simulink model "Scenario_2_power_system_modeling"  (R2023b)
settings: Solver=ode4  StartTime=0.0  StopTime=90  FixedStep=0.01  RelTol=1e-3
values from neighbouring files (symbols this model uses):
  a12 = -1    [simulation_3_Area_scenario.m]    (also in simulation_scenario_1_2_3.m)
  B1 = (1/Rtotal_1) + D1    (= 20.9)    [simulation_3_Area_scenario.m]    (also in simulation_scenario_1_2_3.m = 40.9)
  B2 = (1/Rtotal_2) + D2    (= 21.5)    [simulation_3_Area_scenario.m]    (also in simulation_scenario_1_2_3.m = 41.5)
  D1 = 0.9    [simulation_3_Area_scenario.m]    (also in simulation_scenario_1_2_3.m)
  D2 = 1.5    [simulation_3_Area_scenario.m]    (also in simulation_scenario_1_2_3.m)
  Fhp = 0.4    [simulation_3_Area_scenario.m]    (also in simulation_scenario_1_2_3.m)
  H1 = H1_values(i)    [simulation_3_Area_scenario.m]    (also in simulation_scenario_1_2_3.m)
  H2 = H2_values(i)    [simulation_3_Area_scenario.m]    (also in simulation_scenario_1_2_3.m)
  KI1 = 0.25    [simulation_3_Area_scenario.m]    (also in simulation_scenario_1_2_3.m)
  KI2 = 0.25    [simulation_3_Area_scenario.m]    (also in simulation_scenario_1_2_3.m)
  KI3 = 0.25    [simulation_3_Area_scenario.m]    (also in simulation_scenario_1_2_3.m)
  KI4 = 0.25    [simulation_3_Area_scenario.m]    (also in simulation_scenario_1_2_3.m)
  R1 = 0.1    [simulation_3_Area_scenario.m]    (also in simulation_scenario_1_2_3.m = 0.05)
  R2 = 0.1    [simulation_3_Area_scenario.m]    (also in simulation_scenario_1_2_3.m = 0.05)
  R3 = 0.1    [simulation_3_Area_scenario.m]    (also in simulation_scenario_1_2_3.m = 0.05)
  R4 = 0.1    [simulation_3_Area_scenario.m]    (also in simulation_scenario_1_2_3.m = 0.05)
  Rp = 0.05    [simulation_3_Area_scenario.m]    (also in simulation_scenario_1_2_3.m)
  Rt = 0.38    [simulation_3_Area_scenario.m]    (also in simulation_scenario_1_2_3.m)
  T12 = 2    [simulation_3_Area_scenario.m]    (also in simulation_scenario_1_2_3.m)
  Tch1 = 0.39    [simulation_3_Area_scenario.m]    (also in simulation_scenario_1_2_3.m)
  Tch2 = 0.5    [simulation_3_Area_scenario.m]    (also in simulation_scenario_1_2_3.m)
  Tg1 = 0.23    [simulation_3_Area_scenario.m]    (also in simulation_scenario_1_2_3.m)
  Tg2 = 0.14    [simulation_3_Area_scenario.m]    (also in simulation_scenario_1_2_3.m)
  Tg3 = 0.4    [simulation_3_Area_scenario.m]    (also in simulation_scenario_1_2_3.m)
  Tg4 = 0.3    [simulation_3_Area_scenario.m]    (also in simulation_scenario_1_2_3.m)
  Tr = 5    [simulation_3_Area_scenario.m]    (also in simulation_scenario_1_2_3.m)
  Trh = 7    [simulation_3_Area_scenario.m]    (also in simulation_scenario_1_2_3.m)
  Tw = 2.25    [simulation_3_Area_scenario.m]    (also in simulation_scenario_1_2_3.m)
libraries: dspfdesign x2, simulink x2
settings Model: Creator=themi  LastModifiedBy=themi

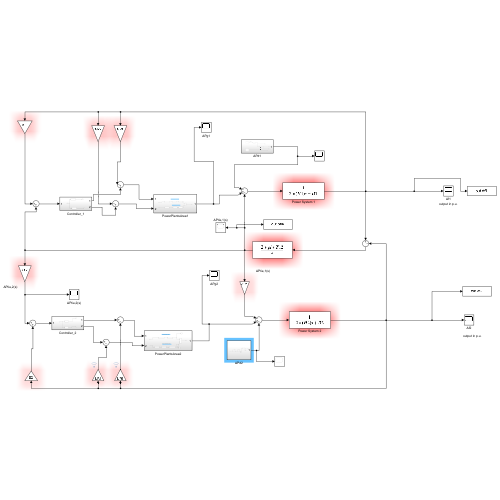
[thumbnail: Simulink's stored preview of the top-level diagram]
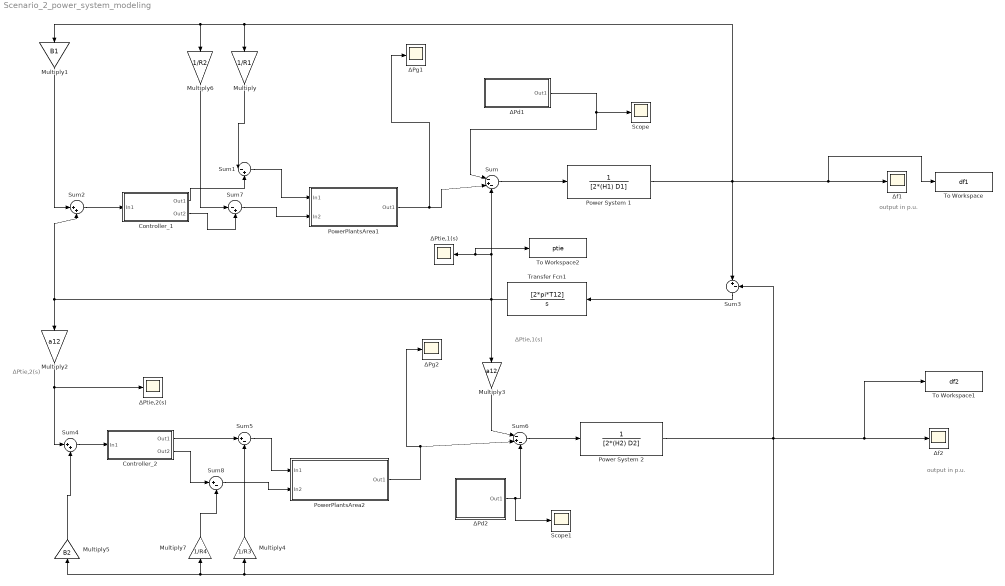
== system Scenario_2_power_system_modeling ==
  note: output in p.u.
  note: output in p.u.
  note: ΔPtie,1(s)
  note: ΔPtie,2(s)
  Controller_1 : Subsystem
  Controller_2 : Subsystem
  Multiply : Gain  Gain=1/R1
  Multiply1 : Gain  Gain=B1
  Multiply2 : Gain  Gain=a12
  Multiply3 : Gain  Gain=a12
  Multiply4 : Gain  Gain=1/R3
  Multiply5 : Gain  Gain=B2
  Multiply6 : Gain  Gain=1/R2
  Multiply7 : Gain  Gain=1/R4
  Power System 1 : TransferFcn  Denominator=[2*(H1) D1]
  Power System 2 : TransferFcn  Denominator=[2*(H2) D2]
  PowerPlantsArea1 : Subsystem
  PowerPlantsArea2 : Subsystem
  Scope : Scope
  Scope1 : Scope
  Sum : Sum  Inputs=|-+-
  Sum1 : Sum  Inputs=|-+
  Sum2 : Sum  Inputs=|++
  Sum3 : Sum  Inputs=|+-
  Sum4 : Sum  Inputs=|++
  Sum5 : Sum  Inputs=|+-
  Sum6 : Sum  Inputs=|-+-
  Sum7 : Sum  Inputs=|-+
  Sum8 : Sum  Inputs=|+-
  To Workspace : ToWorkspace  VariableName=df1  SaveFormat=Structure With Time  SampleTime=-1
  To Workspace1 : ToWorkspace  VariableName=df2  SaveFormat=Structure With Time  SampleTime=-1
  To Workspace2 : ToWorkspace  VariableName=ptie  SaveFormat=Structure With Time  SampleTime=-1
  Transfer Fcn1 : TransferFcn  Numerator=[2*pi*T12]  Denominator=[1 0]
  ΔPd1 : Subsystem
  ΔPd2 : Subsystem
  ΔPg1 : Scope
  ΔPg2 : Scope
  ΔPtie,1(s) : Scope
  ΔPtie,2(s) : Scope
  Δf1 : Scope
  Δf2 : Scope
  wires:
  Sum3/1 -> Transfer Fcn1/1
  Multiply5/1 -> Sum4/2
  Sum/1 -> Power System 1/1
  Multiply4/1 -> Sum5/2
  Sum6/1 -> Power System 2/1
  Sum4/1 -> Controller_2/1(In1)
  Multiply7/1 -> Sum8/2
  Power System 1/1 -> Multiply6/1, Multiply1/1, Multiply/1, To Workspace/1, Δf1/1, Sum3/1
  Multiply3/1 -> Sum6/1
  Sum2/1 -> Controller_1/1(In1)
  Power System 2/1 -> To Workspace1/1, Δf2/1, Multiply7/1, Multiply5/1, Multiply4/1, Sum3/2
  Multiply2/1 -> ΔPtie,2(s)/1, Sum4/1
  Multiply1/1 -> Sum2/1
  Controller_2/1(Out1) -> Sum5/1
  Transfer Fcn1/1 -> Sum2/2, Multiply2/1, Multiply3/1, To Workspace2/1, ΔPtie,1(s)/1, Sum/3
  Multiply/1 -> Sum1/1
  Controller_2/2(Out2) -> Sum8/1
  Controller_1/2(Out2) -> Sum7/2
  Controller_1/1(Out1) -> Sum1/2
  Multiply6/1 -> Sum7/1
  Sum5/1 -> PowerPlantsArea2/1(In1)
  Sum8/1 -> PowerPlantsArea2/2(In2)
  PowerPlantsArea2/1(Out1) -> Sum6/2, ΔPg2/1
  Sum1/1 -> PowerPlantsArea1/1(In1)
  Sum7/1 -> PowerPlantsArea1/2(In2)
  PowerPlantsArea1/1(Out1) -> ΔPg1/1, Sum/2
  ΔPd1/1(Out1) -> Scope/1, Sum/1
  ΔPd2/1(Out1) -> Scope1/1, Sum6/3

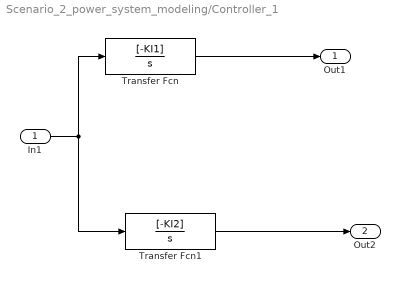
== system Scenario_2_power_system_modeling/Controller_1 ==
  In1 : Inport
  Transfer Fcn : TransferFcn  Numerator=[-KI1]  Denominator=[1 0]
  Transfer Fcn1 : TransferFcn  Numerator=[-KI2]  Denominator=[1 0]
  Out1 : Outport
  Out2 : Outport  Port=2
  wires:
  In1/1 -> Transfer Fcn/1, Transfer Fcn1/1
  Transfer Fcn/1 -> Out1/1
  Transfer Fcn1/1 -> Out2/1

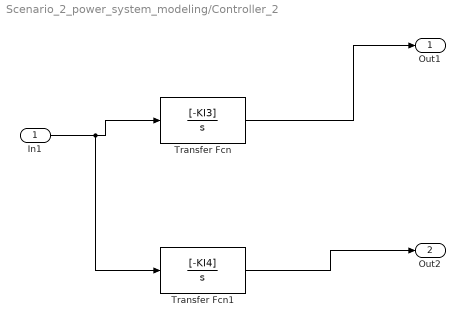
== system Scenario_2_power_system_modeling/Controller_2 ==
  In1 : Inport
  Transfer Fcn : TransferFcn  Numerator=[-KI3]  Denominator=[1 0]
  Transfer Fcn1 : TransferFcn  Numerator=[-KI4]  Denominator=[1 0]
  Out1 : Outport
  Out2 : Outport  Port=2
  wires:
  In1/1 -> Transfer Fcn1/1, Transfer Fcn/1
  Transfer Fcn/1 -> Out1/1
  Transfer Fcn1/1 -> Out2/1

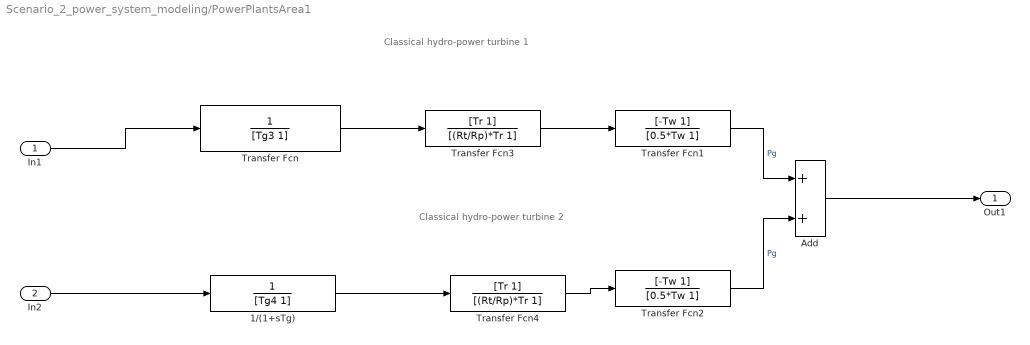
== system Scenario_2_power_system_modeling/PowerPlantsArea1 ==
  note: Classical hydro-power turbine 1
  note: Classical hydro-power turbine 2
  In1 : Inport
  In2 : Inport  Port=2
  1/(1+sTg) : TransferFcn  Denominator=[Tg4 1]
  Add : Sum
  Transfer Fcn : TransferFcn  Denominator=[Tg3 1]
  Transfer Fcn1 : TransferFcn  Numerator=[-Tw 1]  Denominator=[0.5*Tw 1]
  Transfer Fcn2 : TransferFcn  Numerator=[-Tw 1]  Denominator=[0.5*Tw 1]
  Transfer Fcn3 : TransferFcn  Numerator=[Tr 1]  Denominator=[(Rt/Rp)*Tr 1]
  Transfer Fcn4 : TransferFcn  Numerator=[Tr 1]  Denominator=[(Rt/Rp)*Tr 1]
  Out1 : Outport
  wires:
  Transfer Fcn3/1 -> Transfer Fcn1/1
  Transfer Fcn1/1 -> Add/1  "Pg"
  Transfer Fcn/1 -> Transfer Fcn3/1
  In1/1 -> Transfer Fcn/1
  Add/1 -> Out1/1
  In2/1 -> 1/(1+sTg)/1
  Transfer Fcn4/1 -> Transfer Fcn2/1
  1/(1+sTg)/1 -> Transfer Fcn4/1
  Transfer Fcn2/1 -> Add/2  "Pg"

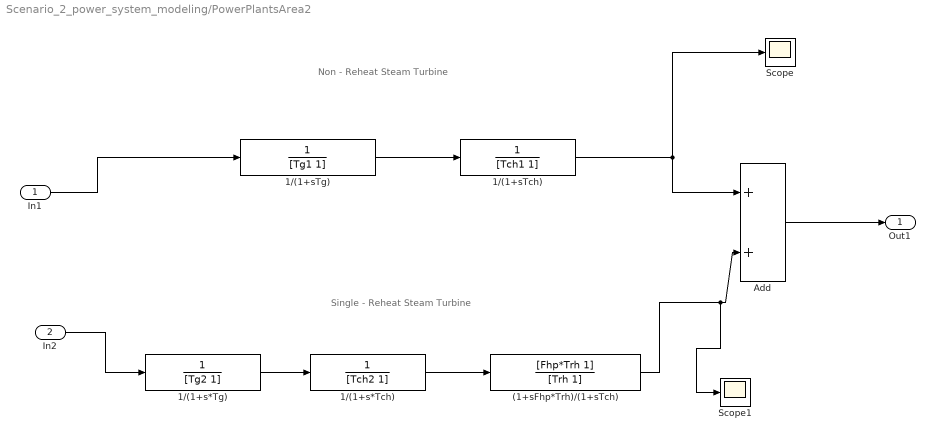
== system Scenario_2_power_system_modeling/PowerPlantsArea2 ==
  note: Non - Reheat Steam Turbine
  note: Single - Reheat Steam Turbine
  In1 : Inport
  In2 : Inport  Port=2
  (1+sFhp*Trh)/(1+sTch) : TransferFcn  Numerator=[Fhp*Trh 1]  Denominator=[Trh 1]
  1/(1+s*Tch) : TransferFcn  Denominator=[Tch2 1]
  1/(1+s*Tg) : TransferFcn  Denominator=[Tg2 1]
  1/(1+sTch) : TransferFcn  Denominator=[Tch1 1]
  1/(1+sTg) : TransferFcn  Denominator=[Tg1 1]
  Add : Sum
  Scope : Scope
  Scope1 : Scope
  Out1 : Outport
  wires:
  In1/1 -> 1/(1+sTg)/1
  1/(1+sTg)/1 -> 1/(1+sTch)/1
  1/(1+s*Tg)/1 -> 1/(1+s*Tch)/1
  1/(1+s*Tch)/1 -> (1+sFhp*Trh)/(1+sTch)/1
  Add/1 -> Out1/1
  1/(1+sTch)/1 -> Scope/1, Add/1
  (1+sFhp*Trh)/(1+sTch)/1 -> Scope1/1, Add/2
  In2/1 -> 1/(1+s*Tg)/1

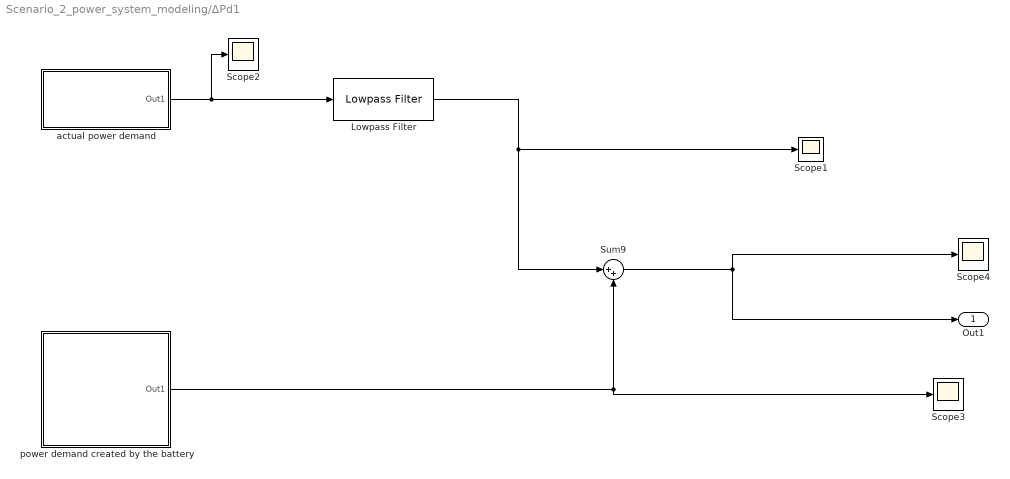
== system Scenario_2_power_system_modeling/ΔPd1 ==
  Lowpass Filter : dspfdesign/Lowpass Filter  FilterType=FIR  DesignForMinimumOrder=on  FilterOrder=50  PassbandFrequency=1  StopbandFrequency=5  PassbandRipple=0.1  StopbandAttenuation=80  SampleRateMode=Specify on dialog  SampleRate=100  SimulateUsing=Interpreted execution  roundingMode=Floor  coeffsDataTypeStr=fixdt(1,16)
  Scope{1..4} (4 alike) : Scope
  Sum9 : Sum  Inputs=|++
  actual power demand : Subsystem
  power demand created by the battery : Subsystem
      mask Display: image('5998565.png');
  Out1 : Outport
  wires:
  Sum9/1 -> Scope4/1, Out1/1
  power demand created by the battery/1(Out1) -> Scope3/1, Sum9/2
  actual power demand/1(Out1) -> Scope2/1, Lowpass Filter/1
  Lowpass Filter/1 -> Scope1/1, Sum9/1

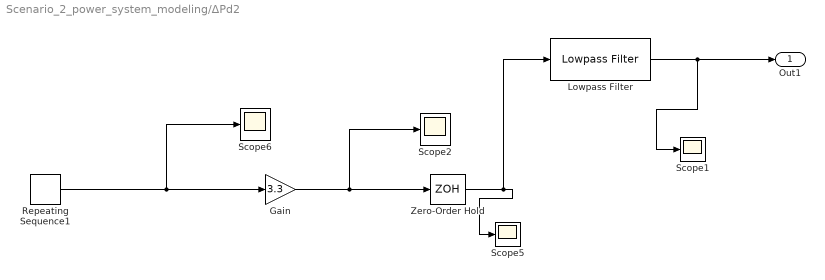
== system Scenario_2_power_system_modeling/ΔPd2 ==
  Gain : Gain  Gain=3.3
  Lowpass Filter : dspfdesign/Lowpass Filter  FilterType=FIR  DesignForMinimumOrder=on  FilterOrder=50  PassbandFrequency=1  StopbandFrequency=5  PassbandRipple=0.1  StopbandAttenuation=80  SampleRateMode=Specify on dialog  SampleRate=100  SimulateUsing=Interpreted execution  roundingMode=Floor  coeffsDataTypeStr=fixdt(1,16)
  Repeating Sequence1 : simulink/Sources/Repeating Sequence  rep_seq_t=t  rep_seq_y=disturbance2
  Scope{1..2,5..6} (4 alike) : Scope
  Zero-Order Hold : ZeroOrderHold  SampleTime=0.01
  Out1 : Outport
  wires:
  Gain/1 -> Scope2/1, Zero-Order Hold/1
  Zero-Order Hold/1 -> Lowpass Filter/1, Scope5/1
  Repeating Sequence1/1 -> Scope6/1, Gain/1
  Lowpass Filter/1 -> Scope1/1, Out1/1

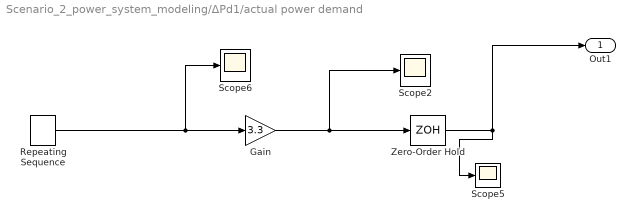
== system Scenario_2_power_system_modeling/ΔPd1/actual power demand ==
  Gain : Gain  Gain=3.3
  Repeating Sequence : simulink/Sources/Repeating Sequence  rep_seq_t=t  rep_seq_y=disturbance1
  Scope2 : Scope
  Scope5 : Scope
  Scope6 : Scope
  Zero-Order Hold : ZeroOrderHold  SampleTime=0.01
  Out1 : Outport
  wires:
  Gain/1 -> Scope2/1, Zero-Order Hold/1
  Repeating Sequence/1 -> Scope6/1, Gain/1
  Zero-Order Hold/1 -> Out1/1, Scope5/1

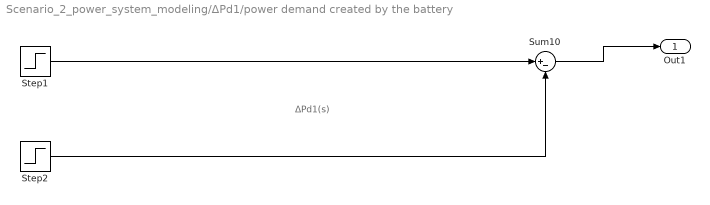
== system Scenario_2_power_system_modeling/ΔPd1/power demand created by the battery ==
  note: ΔPd1(s)
  Step1 : Step  Time=20  After=0.01  SampleTime=0
  Step2 : Step  Time=40  After=0.01  SampleTime=0
  Sum10 : Sum  Inputs=|+-
  Out1 : Outport
  wires:
  Step2/1 -> Sum10/2
  Step1/1 -> Sum10/1
  Sum10/1 -> Out1/1
